simulink model "myo_sfun_one_myo"  (R2013a)
settings: Solver=ode3  StartTime=0.0  StopTime=inf  FixedStep=0.005  RelTol=1e-3
libraries: rtwinlib x1, myo_lib x1
settings Model: Creator=Mark Tomaszewski  LastModifiedBy=Mark Tomaszewski
settings GRTTargetCC: ExtMode=on

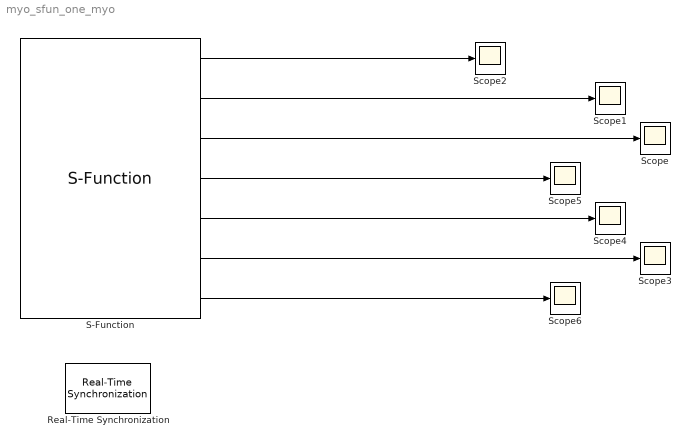
== system myo_sfun_one_myo ==
  Real-Time Synchronization : rtwinlib/Real-Time Synchronization  SampleTime=0.005  MaxMissedTicks=200  ShowMissedTicks=off  YieldWhenWaiting=off
  S-Function : myo_lib/S-Function  emgEnabled=1  countMyos=1
  Scope{,1..6} (7 alike) : Scope
      Scope1 settings: YMin=-750  YMax=1750
      Scope2 settings: YMin=-0.5  YMax=1  SaveName=ScopeData2
      Scope3 settings: SaveName=ScopeData3
      Scope4 settings: SaveName=ScopeData4
      Scope5 settings: SaveName=ScopeData5
      Scope6 settings: YMin=-150  YMax=150  SaveName=ScopeData6
  wires:
  S-Function/1 -> Scope2/1
  S-Function/2 -> Scope1/1
  S-Function/3 -> Scope/1
  S-Function/4 -> Scope5/1
  S-Function/5 -> Scope4/1
  S-Function/6 -> Scope3/1
  S-Function/7 -> Scope6/1
